simulink model "simulacao_unid_2"  (R2015a)
settings: Solver=ode45  SolverMode=SingleTasking  StartTime=0.0  StopTime=600  RelTol=1e-3
settings Model: CovMetricSettings=dwe  CovHtmlReporting=off  covSaveCumulativeToWorkspaceVar=off  CovSaveSingleToWorkspaceVar=off  CovExternalEMLEnable=on  Creator=arthu  LastModifiedBy=arthu
settings DataIOCC: LimitDataPoints=off  SaveFormat=Dataset  ReturnWorkspaceOutputs=on
settings DebuggingCC: SFUnexpectedBacktrackingDiag=error  SFNoUnconditionalDefaultTransitionDiag=error
settings HardwareCC: ProdBitPerPointer=64  ProdLargestAtomicFloat=Float  ProdIntDivRoundTo=Zero  ProdEndianess=LittleEndian  ProdHWDeviceType=Specified
settings ModelReferenceCC: PropagateSignalLabelsOutOfModel=on
settings SFSimCC: SimUseLocalCustomCode=on
settings RTWCC: RTWUseLocalCustomCode=on
settings GRTTargetCC: TargetLangStandard=C99 (ISO)  GeneratePreprocessorConditionals=Use local settings

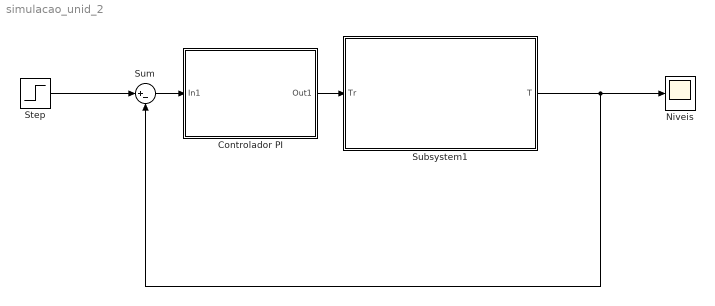
== system simulacao_unid_2 ==
  Controlador PI : Subsystem
  Niveis : Scope
      settings: TimeRange=240  ShowLegends=on  LimitDataPoints=on  MaxDataPoints=500000  SaveName=ScopeData  YMin=-0.12478  YMax=1.12306  SampleTime=-1  DataFormat=Array
  Step : Step  SampleTime=0
  Subsystem1 : Subsystem
  Sum : Sum  Inputs=|+-
  wires:
  Step/1 -> Sum/1
  Subsystem1/1(T) -> Sum/2, Niveis/1
  Sum/1 -> Controlador PI/1(In1)
  Controlador PI/1(Out1) -> Subsystem1/1(Tr)

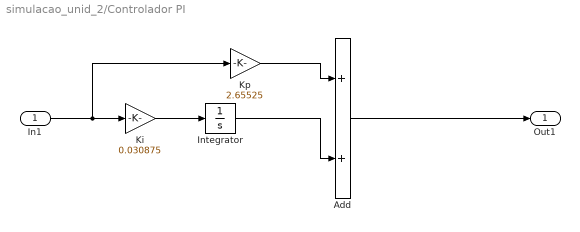
== system simulacao_unid_2/Controlador PI ==
  In1 : Inport
  Add : Sum
  Integrator : Integrator
  Ki : Gain  Gain=0.030875
  Kp : Gain  Gain=2.65525
  Out1 : Outport
  wires:
  Add/1 -> Out1/1
  Kp/1 -> Add/1
  Ki/1 -> Integrator/1
  In1/1 -> Ki/1, Kp/1
  Integrator/1 -> Add/2

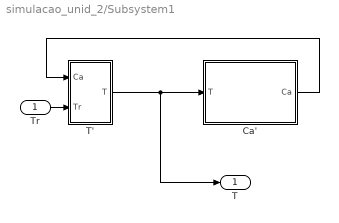
== system simulacao_unid_2/Subsystem1 ==
  Tr : Inport
  Ca' : Subsystem
  T' : Subsystem
  T : Outport
  wires:
  Tr/1 -> T'/2(Tr)
  T'/1(T) -> Ca'/1(T), T/1
  Ca'/1(Ca) -> T'/1(Ca)

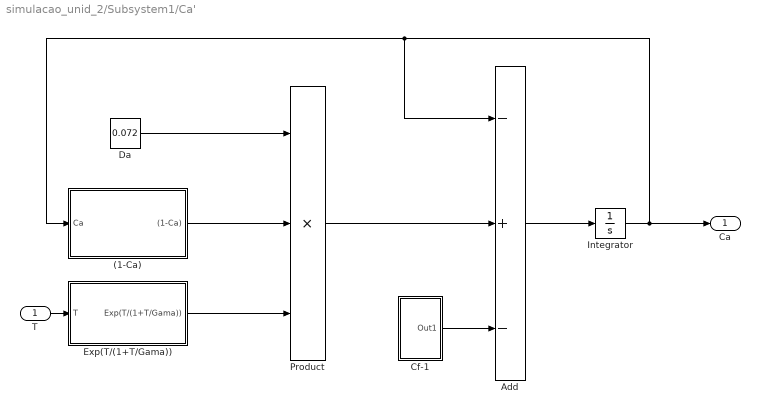
== system simulacao_unid_2/Subsystem1/Ca' ==
  T : Inport
  (1-Ca) : Subsystem
  Add : Sum  Inputs=-+-
  Cf-1 : Subsystem
  Da : Constant  Value=0.072
  Exp(T/(1+T/Gama)) : Subsystem
  Integrator : Integrator
  Product : Product  Inputs=3
  Ca : Outport
  wires:
  Da/1 -> Product/1
  T/1 -> Exp(T/(1+T/Gama))/1(T)
  Cf-1/1(Out1) -> Add/3
  Product/1 -> Add/2
  Add/1 -> Integrator/1
  (1-Ca)/1((1-Ca)) -> Product/2
  Integrator/1 -> (1-Ca)/1(Ca), Add/1, Ca/1
  Exp(T/(1+T/Gama))/1(Exp(T/(1+T/Gama))) -> Product/3

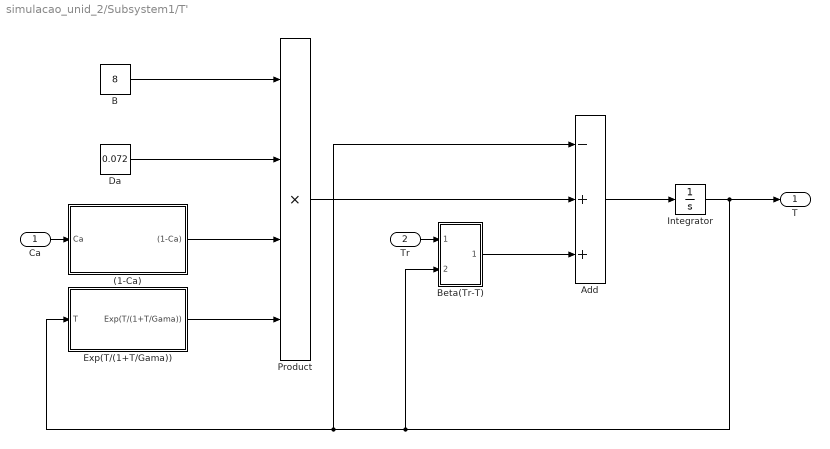
== system simulacao_unid_2/Subsystem1/T' ==
  Ca : Inport
  Tr : Inport  Port=2
  (1-Ca) : Subsystem
  Add : Sum  Inputs=-++
  B : Constant  Value=8
  Beta(Tr-T) : Subsystem
  Da : Constant  Value=0.072
  Exp(T/(1+T/Gama)) : Subsystem
  Integrator : Integrator
  Product : Product  Inputs=4
  T : Outport
  wires:
  Ca/1 -> (1-Ca)/1(Ca)
  Tr/1 -> Beta(Tr-T)/1(In1)
  (1-Ca)/1((1-Ca)) -> Product/3
  Integrator/1 -> Exp(T/(1+T/Gama))/1(T), Add/1, Beta(Tr-T)/2(In2), T/1
  Da/1 -> Product/2
  Exp(T/(1+T/Gama))/1(Exp(T/(1+T/Gama))) -> Product/4
  Product/1 -> Add/2
  B/1 -> Product/1
  Beta(Tr-T)/1(Out1) -> Add/3
  Add/1 -> Integrator/1

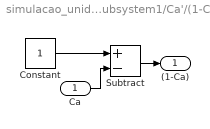
== system simulacao_unid_2/Subsystem1/Ca'/(1-Ca) ==
  Ca : Inport
  Constant : Constant
  Subtract : Sum  Inputs=+-
  (1-Ca) : Outport
  wires:
  Ca/1 -> Subtract/2
  Subtract/1 -> (1-Ca)/1
  Constant/1 -> Subtract/1

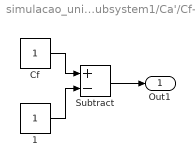
== system simulacao_unid_2/Subsystem1/Ca'/Cf-1 ==
  1 : Constant
  Cf : Constant
  Subtract : Sum  Inputs=+-
  Out1 : Outport
  wires:
  Subtract/1 -> Out1/1
  1/1 -> Subtract/2
  Cf/1 -> Subtract/1

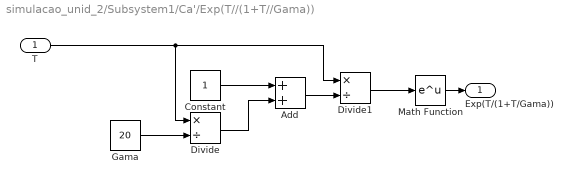
== system simulacao_unid_2/Subsystem1/Ca'/Exp(T//(1+T//Gama)) ==
  T : Inport
  Add : Sum
  Constant : Constant
  Divide : Product  Inputs=*/
  Divide1 : Product  Inputs=*/
  Gama : Constant  Value=20
  Math Function : Math  SaturateOnIntegerOverflow=on
  Exp(T/(1+T/Gama)) : Outport
  wires:
  Gama/1 -> Divide/2
  Constant/1 -> Add/1
  Divide1/1 -> Math Function/1
  Add/1 -> Divide1/2
  Divide/1 -> Add/2
  Math Function/1 -> Exp(T/(1+T/Gama))/1
  T/1 -> Divide1/1, Divide/1

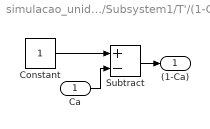
== system simulacao_unid_2/Subsystem1/T'/(1-Ca) ==
  Ca : Inport
  Constant : Constant
  Subtract : Sum  Inputs=+-
  (1-Ca) : Outport
  wires:
  Ca/1 -> Subtract/2
  Subtract/1 -> (1-Ca)/1
  Constant/1 -> Subtract/1

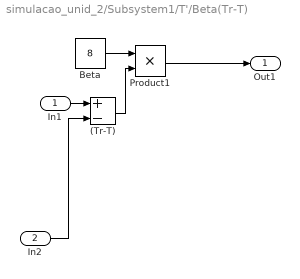
== system simulacao_unid_2/Subsystem1/T'/Beta(Tr-T) ==
  In1 : Inport
  In2 : Inport  Port=2
  (Tr-T) : Sum  Inputs=+-
  Beta : Constant  Value=8
  Product1 : Product
  Out1 : Outport
  wires:
  Product1/1 -> Out1/1
  In2/1 -> (Tr-T)/2
  (Tr-T)/1 -> Product1/2
  Beta/1 -> Product1/1
  In1/1 -> (Tr-T)/1

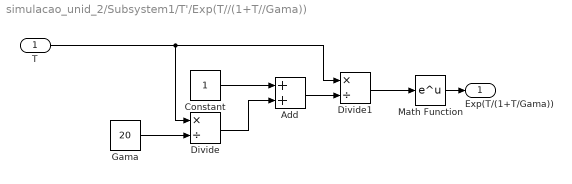
== system simulacao_unid_2/Subsystem1/T'/Exp(T//(1+T//Gama)) ==
  T : Inport
  Add : Sum
  Constant : Constant
  Divide : Product  Inputs=*/
  Divide1 : Product  Inputs=*/
  Gama : Constant  Value=20
  Math Function : Math  SaturateOnIntegerOverflow=on
  Exp(T/(1+T/Gama)) : Outport
  wires:
  Gama/1 -> Divide/2
  Constant/1 -> Add/1
  Divide1/1 -> Math Function/1
  Add/1 -> Divide1/2
  Divide/1 -> Add/2
  Math Function/1 -> Exp(T/(1+T/Gama))/1
  T/1 -> Divide1/1, Divide/1
